simulink model "hdv_ctrl_2021_08_12"  (R2020a)
settings: Solver=ode23tb  StartTime=0.0  StopTime=simulation_length  MaxStep=tsample
values from neighbouring files (symbols this model uses):
  available_torque = [-660.07, -796.01, -907.96, -1019.98, -1070.98, -1123.89,     -1175.99, -1224.03, -1254.98, -1250.99, -1250.98, -1250.98, -1050.04,     -934.05, -780.06, -650, -450, -350, 350, 450, 650, 780.06, 934.05,     1050.04, 1250.98, 1250.98, 1250.99, 1254.98, 1224.03, 1175.99,     1123.89, 1070.98, 1019.98, 907.96, 796.01, 660.07]    [control_design.m]
  d1_ff = d1_ff_temp    (= 1.95205196931)    [control_design.m]
  d2_ff = d2_ff_temp    (= 1.95205196931)    [control_design.m]
  ki_ctrl_diff_speed = 4/n2    (= 4)    [control_design.m]
  ki_ctrl_sum_speed = 4/n1    (= 4)    [control_design.m]
  kp_ctrl_diff_speed = 0.25/n2    (= 0.25)    [control_design.m]
  kp_ctrl_sum_speed = 0.25/n1    (= 0.25)    [control_design.m]
  omega_e_rpm_ref = 1940    [control_design.m]
  omega_l_1_ref_rpm = v_track1_ref/3.6/R_tg/(2*pi)*60    (= 48.1674665855)    [control_design.m]
  omega_l_2_ref_rpm = v_track2_ref/3.6/R_tg/(2*pi)*60    (= 48.1674665855)    [control_design.m]
  omega_l_max_rpm = omega_l_max/(2*pi)*60    (= 66.2302665551)    [control_design.m]
  R_tg = 0.44056    [control_design.m]
  rpm = [-2140, -2100, -2000, -1900, -1800, -1700, -1600, -1500, -1400,          -1300, -1200, -1100, -1000, -900, -800, -700, -600, -5, 5, 600,          700, 800, 900, 1000, 1100, 1200, 1300, 1400, 1500, 1600, 1700, 1800,         1900, 2000, 2100, 2140]    [control_design.m]
  simulation_length = 45    [control_design.m]
  tau_load = -1200*41.4    (= -49680)    [control_design.m]
  tau_load_max = 1600*41.4    (= 66240)    [control_design.m]
  tsample = 1e-3    (= 0.001)    [control_design.m]
  v_track1_ref = 8    [control_design.m]
  v_track2_ref = 8    [control_design.m]
libraries: nesl_utility x24, fl_lib x13, linear_swashplate_ctrl_lib x4, variable_displacement_motor_lib x2, variable_displacement_pump_lib x2, flexshaft_lib x2, gear_lib x2, simulink x2, engine_speed_ctrl_lib x1, Liebherr_Engine_D934_lib x1
settings Model: SimulationMode=accelerator  Creator=dbagn  LastModifiedBy=dbagn
settings DataIOCC: ReturnWorkspaceOutputs=off

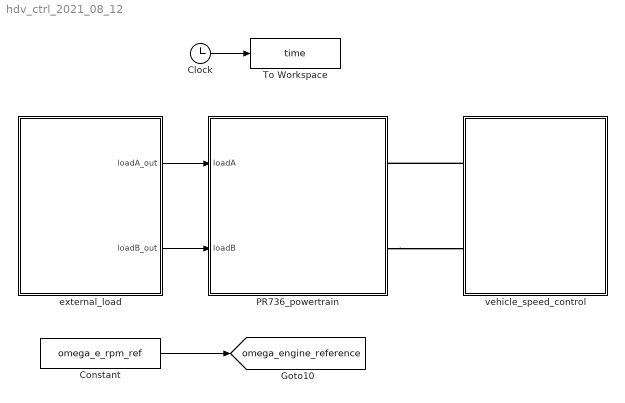
== system hdv_ctrl_2021_08_12 ==
  Clock : Clock
  Constant : Constant  Value=omega_e_rpm_ref
  PR736_powertrain : Subsystem
  To Workspace : ToWorkspace  VariableName=time  SampleTime=tsample
      settings: MaxDataPoints=Nsample
  external_load : Subsystem
  vehicle_speed_control : Subsystem
  tag scope: omega_engine_reference=global
  wires:
  Clock/1 -> To Workspace/1
  Constant/1 -> [omega_engine_reference]
  external_load/2(loadB_out) -> PR736_powertrain/2(loadB)
  external_load/1(loadA_out) -> PR736_powertrain/1(loadA)
  connections:
  vehicle_speed_control/LConn1 -- PR736_powertrain/RConn1
  PR736_powertrain/RConn2 -- vehicle_speed_control/LConn2

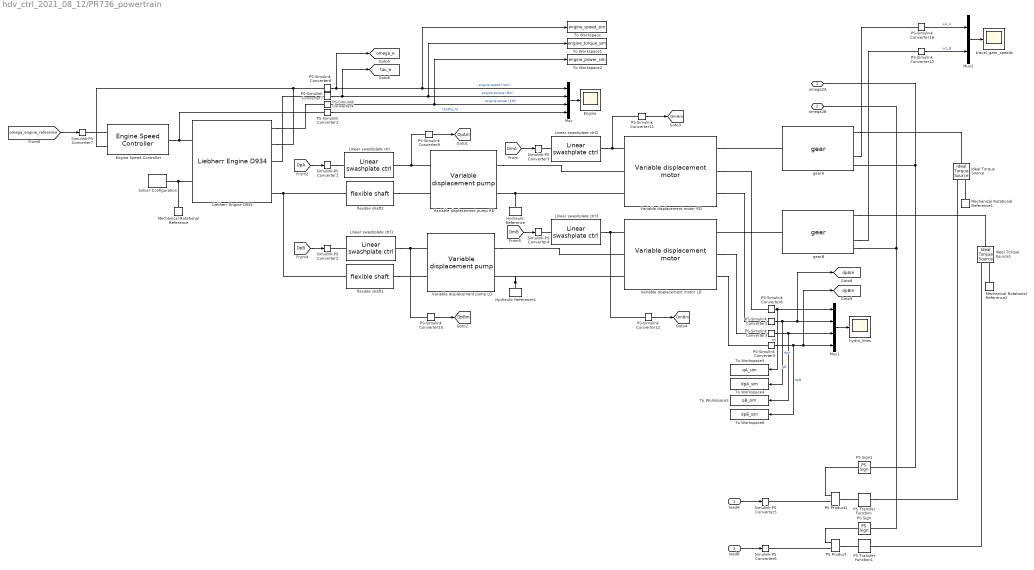
== system hdv_ctrl_2021_08_12/PR736_powertrain ==
  loadA : Inport
  loadB : Inport  Port=2
  Engine : Scope
  Engine Speed Controller : engine_speed_ctrl_lib/Engine Speed Controller  kp=0.25 s  kint=2  kd=0 s^2  t_out_specify=off  t_out_priority=None  t_out=0  t_out_nominal_specify=off  t_out_nominal_unit=1  t_out_nominal_value=1
      settings: InternalSimscapePortConfiguration="{\"Bottom\":[],\"Left\":[{\"id\":\"we_ref\",\"label\":\"we_ref\",\"type\":\"input\"},{\"id\":\"we\",\"label\":\"we\",\"type\":\"input\"}],\"Right\":[{\"id\":\"theta\",\"label\":\"tS\",\"type\":\"output\"}],\"Top\":[]}"
  Hydraulic Reference : fl_lib/Hydraulic/Hydraulic Elements/Hydraulic Reference
  Hydraulic Reference1 : fl_lib/Hydraulic/Hydraulic Elements/Hydraulic Reference
  Ideal Torque Source : fl_lib/Mechanical/Mechanical Sources/Ideal Torque Source
  Ideal Torque Source1 : fl_lib/Mechanical/Mechanical Sources/Ideal Torque Source
  Liebherr Engine D934 : Liebherr_Engine_D934_lib/Liebherr Engine D934  dynamic_response=simscape.enum.onoff.on  cshaft_inertia=7.5 kg*m^2  initial_speed=5
      settings: InternalSimscapePortConfiguration="{\"Bottom\":[],\"Left\":[{\"id\":\"tS\",\"label\":\"tS\",\"type\":\"input\"},{\"id\":\"C\",\"label\":\"C\",\"type\":\"foundation.mechanical.rotational.rotational\"}],\"Right\":[{\"id\":\"PE\",\"label\":\"PE\",\"type\":\"output\"},{\"id\":\"wE\",\"label\":\"wE\",\"type\":\"output\"},{\"id\":\"tE\",\"label\":\"tE\",\"type\":\"output\"},{\"id\":\"eE\",\"label\":\"eE\",\"type\":\"output\"},{\"id\":\"D\",\"label\":\"D\",\"type\":\"foundation.mechanical.rotational.rotational\"}],\"Top\":[]}"
  Linear swashplate ctrl : linear_swashplate_ctrl_lib/Linear swashplate ctrl  a12=1 1/s  b2=1 1/m/s  k1=100 m  k2=20.5 m  N=10 m  kv=10  xv_specify=off  xv_priority=None  xv=0 m  xv_nominal_specify=off  xv_nominal_unit=m  xv_nominal_value=1  D1_specify=off  D1_priority=None  D1=0  D1_nominal_specify=off  D1_nominal_unit=1  D1_nominal_value=1  D2_specify=off  D2_priority=None  D2=0  D2_nominal_specify=off  D2_nominal_unit=1  D2_nominal_value=1
      settings: InternalSimscapePortConfiguration="{\"Bottom\":[],\"Left\":[{\"id\":\"D_ref\",\"label\":\"Dref\",\"type\":\"input\"}],\"Right\":[{\"id\":\"Dout\",\"label\":\"Dout\",\"type\":\"output\"}],\"Top\":[]}"
  Linear swashplate ctrl1 : linear_swashplate_ctrl_lib/Linear swashplate ctrl  a12=1 1/s  b2=1 1/m/s  k1=100 m  k2=20.5 m  N=10 m  kv=10  xv_specify=off  xv_priority=None  xv=0 m  xv_nominal_specify=off  xv_nominal_unit=m  xv_nominal_value=1  D1_specify=off  D1_priority=None  D1=0  D1_nominal_specify=off  D1_nominal_unit=1  D1_nominal_value=1  D2_specify=off  D2_priority=None  D2=0  D2_nominal_specify=off  D2_nominal_unit=1  D2_nominal_value=1
      settings: InternalSimscapePortConfiguration="{\"Bottom\":[],\"Left\":[{\"id\":\"D_ref\",\"label\":\"Dref\",\"type\":\"input\"}],\"Right\":[{\"id\":\"Dout\",\"label\":\"Dout\",\"type\":\"output\"}],\"Top\":[]}"
  Linear swashplate ctrl2 : linear_swashplate_ctrl_lib/Linear swashplate ctrl  a12=1 1/s  b2=1 1/m/s  k1=100 m  k2=20.5 m  N=5 m  kv=20  xv_specify=off  xv_priority=None  xv=0 m  xv_nominal_specify=off  xv_nominal_unit=m  xv_nominal_value=1  D1_specify=off  D1_priority=None  D1=0  D1_nominal_specify=off  D1_nominal_unit=1  D1_nominal_value=1  D2_specify=off  D2_priority=None  D2=0  D2_nominal_specify=off  D2_nominal_unit=1  D2_nominal_value=1
      settings: InternalSimscapePortConfiguration="{\"Bottom\":[],\"Left\":[{\"id\":\"D_ref\",\"label\":\"Dref\",\"type\":\"input\"}],\"Right\":[{\"id\":\"Dout\",\"label\":\"Dout\",\"type\":\"output\"}],\"Top\":[]}"
  Linear swashplate ctrl3 : linear_swashplate_ctrl_lib/Linear swashplate ctrl  a12=1 1/s  b2=1 1/m/s  k1=100 m  k2=20.5 m  N=5 m  kv=20  xv_specify=off  xv_priority=None  xv=0 m  xv_nominal_specify=off  xv_nominal_unit=m  xv_nominal_value=1  D1_specify=off  D1_priority=None  D1=0  D1_nominal_specify=off  D1_nominal_unit=1  D1_nominal_value=1  D2_specify=off  D2_priority=None  D2=0  D2_nominal_specify=off  D2_nominal_unit=1  D2_nominal_value=1
      settings: InternalSimscapePortConfiguration="{\"Bottom\":[],\"Left\":[{\"id\":\"D_ref\",\"label\":\"Dref\",\"type\":\"input\"}],\"Right\":[{\"id\":\"Dout\",\"label\":\"Dout\",\"type\":\"output\"}],\"Top\":[]}"
  Mechanical Rotational Reference : fl_lib/Mechanical/Rotational Elements/Mechanical Rotational Reference
  Mechanical Rotational Reference1 : fl_lib/Mechanical/Rotational Elements/Mechanical Rotational Reference
  Mechanical Rotational Reference2 : fl_lib/Mechanical/Rotational Elements/Mechanical Rotational Reference
  Mux : Mux
  Mux1 : Mux
  Mux2 : Mux  Inputs=2
  PS Product : fl_lib/Physical Signals/Functions/PS Product
  PS Product1 : fl_lib/Physical Signals/Functions/PS Product
  PS Sign : fl_lib/Physical Signals/Nonlinear Operators/PS Sign
      settings: SourceProductBaseCode=SS  InternalSimscapePortConfiguration="{\"Bottom\":[],\"Left\":[{\"id\":\"I\",\"label\":\"\",\"type\":\"input\"}],\"Right\":[{\"id\":\"O\",\"label\":\"\",\"type\":\"output\"}],\"Top\":[]}"
  PS Sign1 : fl_lib/Physical Signals/Nonlinear Operators/PS Sign
      settings: SourceProductBaseCode=SS  InternalSimscapePortConfiguration="{\"Bottom\":[],\"Left\":[{\"id\":\"I\",\"label\":\"\",\"type\":\"input\"}],\"Right\":[{\"id\":\"O\",\"label\":\"\",\"type\":\"output\"}],\"Top\":[]}"
  PS Transfer Function : fl_lib/Physical Signals/Linear Operators/PS Transfer Function  transfer_function_type=foundation.enum.transfer_function_type.lag  T=1 s  T1=2 s  T2=1 s  y0=0 N*m
      settings: SourceProductBaseCode=SS  InternalSimscapePortConfiguration="{\"Bottom\":[],\"Left\":[{\"id\":\"U\",\"label\":\"\",\"type\":\"input\"}],\"Right\":[{\"id\":\"Y\",\"label\":\"\",\"type\":\"output\"}],\"Top\":[]}"
  PS Transfer Function1 : fl_lib/Physical Signals/Linear Operators/PS Transfer Function  transfer_function_type=foundation.enum.transfer_function_type.lag  T=1 s  T1=2 s  T2=1 s  y0=0 N*m
      settings: SourceProductBaseCode=SS  InternalSimscapePortConfiguration="{\"Bottom\":[],\"Left\":[{\"id\":\"U\",\"label\":\"\",\"type\":\"input\"}],\"Right\":[{\"id\":\"Y\",\"label\":\"\",\"type\":\"output\"}],\"Top\":[]}"
  PS-Simulink Converter1 : nesl_utility/PS-Simulink Converter  PhysicalDomain=network_engine_domain  SubClassName=ps_output  LeftPortType=input  RightPortType=output  PseudoPeriodic=off  Frequencies=[]  Unit=inherit  AffineConversion=off
  PS-Simulink Converter{2,5,9..12} (6 alike) : nesl_utility/PS-Simulink Converter  PhysicalDomain=network_engine_domain  SubClassName=ps_output  LeftPortType=input  RightPortType=output  PseudoPeriodic=off  Frequencies=[]  Unit=bar  AffineConversion=off
  PS-Simulink Converter13 : nesl_utility/PS-Simulink Converter  PhysicalDomain=network_engine_domain  SubClassName=ps_output  LeftPortType=input  RightPortType=output  PseudoPeriodic=off  Frequencies=[]  Unit=rpm  AffineConversion=on
  PS-Simulink Converter16 : nesl_utility/PS-Simulink Converter  PhysicalDomain=network_engine_domain  SubClassName=ps_output  LeftPortType=input  RightPortType=output  PseudoPeriodic=off  Frequencies=[]  Unit=rpm  AffineConversion=on
  PS-Simulink Converter3 : nesl_utility/PS-Simulink Converter  PhysicalDomain=network_engine_domain  SubClassName=ps_output  LeftPortType=input  RightPortType=output  PseudoPeriodic=off  Frequencies=[]  Unit=l/min  AffineConversion=off
  PS-Simulink Converter4 : nesl_utility/PS-Simulink Converter  PhysicalDomain=network_engine_domain  SubClassName=ps_output  LeftPortType=input  RightPortType=output  PseudoPeriodic=off  Frequencies=[]  Unit=kW  AffineConversion=off
  PS-Simulink Converter6 : nesl_utility/PS-Simulink Converter  PhysicalDomain=network_engine_domain  SubClassName=ps_output  LeftPortType=input  RightPortType=output  PseudoPeriodic=off  Frequencies=[]  Unit=rpm  AffineConversion=off
  PS-Simulink Converter7 : nesl_utility/PS-Simulink Converter  PhysicalDomain=network_engine_domain  SubClassName=ps_output  LeftPortType=input  RightPortType=output  PseudoPeriodic=off  Frequencies=[]  Unit=inherit  AffineConversion=off
  PS-Simulink Converter8 : nesl_utility/PS-Simulink Converter  PhysicalDomain=network_engine_domain  SubClassName=ps_output  LeftPortType=input  RightPortType=output  PseudoPeriodic=off  Frequencies=[]  Unit=l/min  AffineConversion=off
  Simulink-PS Converter{1..4} (4 alike) : nesl_utility/Simulink-PS Converter  PhysicalDomain=network_engine_domain  SubClassName=ps_input  LeftPortType=input  RightPortType=output  PseudoPeriodic=off  Frequencies=[]  NoiseDistribution=none  NoiseParameters=[]  Unit=1  AffineConversion=off  FilteringAndDerivatives=provide  SimscapeFilterOrder=1  InputFilterTimeConstant=0.001  UdotUserProvided=0
  Simulink-PS Converter5 : nesl_utility/Simulink-PS Converter  PhysicalDomain=network_engine_domain  SubClassName=ps_input  LeftPortType=input  RightPortType=output  PseudoPeriodic=off  Frequencies=[]  NoiseDistribution=none  NoiseParameters=[]  Unit=N*m  AffineConversion=off  FilteringAndDerivatives=provide  SimscapeFilterOrder=1  InputFilterTimeConstant=0.001  UdotUserProvided=0
  Simulink-PS Converter6 : nesl_utility/Simulink-PS Converter  PhysicalDomain=network_engine_domain  SubClassName=ps_input  LeftPortType=input  RightPortType=output  PseudoPeriodic=off  Frequencies=[]  NoiseDistribution=none  NoiseParameters=[]  Unit=N*m  AffineConversion=off  FilteringAndDerivatives=provide  SimscapeFilterOrder=1  InputFilterTimeConstant=0.001  UdotUserProvided=0
  Simulink-PS Converter7 : nesl_utility/Simulink-PS Converter  PhysicalDomain=network_engine_domain  SubClassName=ps_input  LeftPortType=input  RightPortType=output  PseudoPeriodic=off  Frequencies=[]  NoiseDistribution=none  NoiseParameters=[]  Unit=rpm  AffineConversion=off  FilteringAndDerivatives=provide  SimscapeFilterOrder=1  InputFilterTimeConstant=0.001  UdotUserProvided=0
  Solver Configuration : nesl_utility/Solver Configuration  PhysicalDomain=network_engine_domain  SubClassName=solver  LeftPortType=input  RightPortType=generic  Tones=[]  Harmonics=[]  SimulateNoise=off  Profile=off  UseLocalSampling=off  EnableSwitchedLinearOptims=on  FrequencyDomain=off  UseCCode=off  RelTol=0.001  AbsTol=1e-06  MinStep=1e-09  ToWorkspace=off  RevertToSquareIcSolve=off  NumHomotopyIterations=100  PhasorMode=off  PhasorModeNumHarmonics=1  DoDC=off  ResidualTolerance=1e-09  UseLocalSolver=on  LocalSolverChoice=NE_BACKWARD_EULER_ADVANCER  LocalSolverSampleTime=tsample  DoFixedCost=on  MaxNonlinIter=3  MaxModeIter=2  LinearAlgebra=auto  EquationFormulation=NE_TIME_EF  DelaysMemoryBudget=1024  AutomaticFiltering=on  FilteringTimeConstant=tsample  PartitionStorageMethod=AS_NEEDED  PartitionMemoryBudget=1024  PartitionMethod=ROBUST
  To Workspace : ToWorkspace  VariableName=engine_speed_sim  SampleTime=tsample
      settings: MaxDataPoints=Nsample
  To Workspace1 : ToWorkspace  VariableName=engine_torque_sim  SampleTime=tsample
      settings: MaxDataPoints=Nsample
  To Workspace2 : ToWorkspace  VariableName=engine_power_sim  SampleTime=tsample
      settings: MaxDataPoints=Nsample
  To Workspace3 : ToWorkspace  VariableName=qA_sim  SampleTime=tsample
      settings: MaxDataPoints=Nsample
  To Workspace4 : ToWorkspace  VariableName=dpA_sim  SampleTime=tsample
      settings: MaxDataPoints=Nsample
  To Workspace5 : ToWorkspace  VariableName=qB_sim  SampleTime=tsample
      settings: MaxDataPoints=Nsample
  To Workspace6 : ToWorkspace  VariableName=dpB_sim  SampleTime=tsample
      settings: MaxDataPoints=Nsample
  Variable displacement motor LD : variable_displacement_motor_lib/Variable displacement motor  max_Dv=Vm_nom cm^3/rev  min_Dv=20 cm^3/rev  inertia_motor=0.0402 kg*m^2  oil_vol=4.1 l  eta_mech=eta_m_m  eta_vol=eta_v_m  t_specify=off  t_priority=None  t=0 N*m  t_nominal_specify=off  t_nominal_unit=N*m  t_nominal_value=1  q_specify=off  q_priority=None  q=0 m^3/s  q_nominal_specify=off  q_nominal_unit=m^3/s  q_nominal_value=1  qt_specify=off  qt_priority=None  qt=0 m^3/s  qt_nominal_specify=off  qt_nominal_unit=m^3/s  qt_nominal_value=1  Dv_specify=off  Dv_priority=None  Dv=0 cm^3/rev  Dv_nominal_specify=off  Dv_nominal_unit=cm^3/rev  Dv_nominal_value=1  dp_specify=off  dp_priority=None  dp=0 Pa  dp_nominal_specify=off  dp_nominal_unit=Pa  dp_nominal_value=1  wm_specify=off  wm_priority=None  wm=0 rad/s  wm_nominal_specify=off  wm_nominal_unit=rad/s  wm_nominal_value=1
      settings: InternalSimscapePortConfiguration="{\"Bottom\":[],\"Left\":[{\"id\":\"Vd\",\"label\":\"Vd\",\"type\":\"input\"},{\"id\":\"A\",\"label\":\"A\",\"type\":\"foundation.hydraulic.hydraulic\"},{\"id\":\"B\",\"label\":\"B\",\"type\":\"foundation.hydraulic.hydraulic\"}],\"Right\":[{\"id\":\"C\",\"label\":\"C\",\"type\":\"foundation.mechanical.rotational.rotational\"},{\"id\":\"q_out\",\"label\":\"q\",\"type\":\"output\"},{\"id\":\"delta_p_out\",\"label\":\"delta_p\",\"type\":\"output\"}],\"Top\":[]}"
  Variable displacement motor RD : variable_displacement_motor_lib/Variable displacement motor  max_Dv=Vm_nom cm^3/rev  min_Dv=20 cm^3/rev  inertia_motor=0.0402 kg*m^2  oil_vol=4.1 l  eta_mech=eta_m_m  eta_vol=eta_v_m  t_specify=off  t_priority=None  t=0 N*m  t_nominal_specify=off  t_nominal_unit=N*m  t_nominal_value=1  q_specify=off  q_priority=None  q=0 m^3/s  q_nominal_specify=off  q_nominal_unit=m^3/s  q_nominal_value=1  qt_specify=off  qt_priority=None  qt=0 m^3/s  qt_nominal_specify=off  qt_nominal_unit=m^3/s  qt_nominal_value=1  Dv_specify=off  Dv_priority=None  Dv=0 cm^3/rev  Dv_nominal_specify=off  Dv_nominal_unit=cm^3/rev  Dv_nominal_value=1  dp_specify=off  dp_priority=None  dp=0 Pa  dp_nominal_specify=off  dp_nominal_unit=Pa  dp_nominal_value=1  wm_specify=off  wm_priority=None  wm=0 rad/s  wm_nominal_specify=off  wm_nominal_unit=rad/s  wm_nominal_value=1
      settings: InternalSimscapePortConfiguration="{\"Bottom\":[],\"Left\":[{\"id\":\"Vd\",\"label\":\"Vd\",\"type\":\"input\"},{\"id\":\"A\",\"label\":\"A\",\"type\":\"foundation.hydraulic.hydraulic\"},{\"id\":\"B\",\"label\":\"B\",\"type\":\"foundation.hydraulic.hydraulic\"}],\"Right\":[{\"id\":\"C\",\"label\":\"C\",\"type\":\"foundation.mechanical.rotational.rotational\"},{\"id\":\"q_out\",\"label\":\"q\",\"type\":\"output\"},{\"id\":\"delta_p_out\",\"label\":\"delta_p\",\"type\":\"output\"}],\"Top\":[]}"
  Variable displacement pump LD : variable_displacement_pump_lib/Variable displacement pump  max_Dv=Vp_nom cm^3/rev  inertia_pump=0.027 kg*m^2  oil_vol=3.0 l  eta_mech=eta_m_p  eta_vol=eta_v_p  t_specify=off  t_priority=None  t=0 N*m  t_nominal_specify=off  t_nominal_unit=N*m  t_nominal_value=1  q_specify=off  q_priority=None  q=0 m^3/s  q_nominal_specify=off  q_nominal_unit=m^3/s  q_nominal_value=1  qt_specify=off  qt_priority=None  qt=0 m^3/s  qt_nominal_specify=off  qt_nominal_unit=m^3/s  qt_nominal_value=1  Dv_specify=off  Dv_priority=None  Dv=0 cm^3/rev  Dv_nominal_specify=off  Dv_nominal_unit=cm^3/rev  Dv_nominal_value=1  dp_specify=off  dp_priority=None  dp=0 Pa  dp_nominal_specify=off  dp_nominal_unit=Pa  dp_nominal_value=1  we_specify=off  we_priority=None  we=0 rad/s  we_nominal_specify=off  we_nominal_unit=rad/s  we_nominal_value=1
      settings: InternalSimscapePortConfiguration="{\"Bottom\":[],\"Left\":[{\"id\":\"Vd\",\"label\":\"Vd\",\"type\":\"input\"},{\"id\":\"C\",\"label\":\"C\",\"type\":\"foundation.mechanical.rotational.rotational\"}],\"Right\":[{\"id\":\"A\",\"label\":\"A\",\"type\":\"foundation.hydraulic.hydraulic\"},{\"id\":\"B\",\"label\":\"B\",\"type\":\"foundation.hydraulic.hydraulic\"}],\"Top\":[]}"
  Variable displacement pump RD : variable_displacement_pump_lib/Variable displacement pump  max_Dv=Vp_nom cm^3/rev  inertia_pump=0.027 kg*m^2  oil_vol=3.0 l  eta_mech=eta_m_p  eta_vol=eta_v_p  t_specify=off  t_priority=None  t=0 N*m  t_nominal_specify=off  t_nominal_unit=N*m  t_nominal_value=1  q_specify=off  q_priority=None  q=0 m^3/s  q_nominal_specify=off  q_nominal_unit=m^3/s  q_nominal_value=1  qt_specify=off  qt_priority=None  qt=0 m^3/s  qt_nominal_specify=off  qt_nominal_unit=m^3/s  qt_nominal_value=1  Dv_specify=off  Dv_priority=None  Dv=0 cm^3/rev  Dv_nominal_specify=off  Dv_nominal_unit=cm^3/rev  Dv_nominal_value=1  dp_specify=off  dp_priority=None  dp=0 Pa  dp_nominal_specify=off  dp_nominal_unit=Pa  dp_nominal_value=1  we_specify=off  we_priority=None  we=0 rad/s  we_nominal_specify=off  we_nominal_unit=rad/s  we_nominal_value=1
      settings: InternalSimscapePortConfiguration="{\"Bottom\":[],\"Left\":[{\"id\":\"Vd\",\"label\":\"Vd\",\"type\":\"input\"},{\"id\":\"C\",\"label\":\"C\",\"type\":\"foundation.mechanical.rotational.rotational\"}],\"Right\":[{\"id\":\"A\",\"label\":\"A\",\"type\":\"foundation.hydraulic.hydraulic\"},{\"id\":\"B\",\"label\":\"B\",\"type\":\"foundation.hydraulic.hydraulic\"}],\"Top\":[]}"
  flexible shaft1 : flexshaft_lib/flexible shaft  b1=b1 N*m/(rad/s)  J1=J1 kg*m^2  b2=b2 N*m/(rad/s)  J2=J2 kg*m^2  b_theta=b_theta N*m/(rad/s)  k_theta=k_theta N*m/rad  w_1_specify=off  w_1_priority=None  w_1=0 rad/s  w_1_nominal_specify=off  w_1_nominal_unit=rad/s  w_1_nominal_value=1  w_2_specify=off  w_2_priority=None  w_2=0 rad/s  w_2_nominal_specify=off  w_2_nominal_unit=rad/s  w_2_nominal_value=1  t_1_specify=off  t_1_priority=None  t_1=0 N*m  t_1_nominal_specify=off  t_1_nominal_unit=N*m  t_1_nominal_value=1  t_2_specify=off  t_2_priority=None  t_2=0 N*m  t_2_nominal_specify=off  t_2_nominal_unit=N*m  t_2_nominal_value=1  t_theta_specify=off  t_theta_priority=None  t_theta=0 N*m  t_theta_nominal_specify=off  t_theta_nominal_unit=N*m  t_theta_nominal_value=1
      settings: InternalSimscapePortConfiguration="{\"Bottom\":[],\"Left\":[{\"id\":\"S1\",\"label\":\"S1\",\"type\":\"foundation.mechanical.rotational.rotational\"}],\"Right\":[{\"id\":\"S2\",\"label\":\"S2\",\"type\":\"foundation.mechanical.rotational.rotational\"}],\"Top\":[]}"
  flexible shaft2 : flexshaft_lib/flexible shaft  b1=b1 N*m/(rad/s)  J1=J1 kg*m^2  b2=b2 N*m/(rad/s)  J2=J2 kg*m^2  b_theta=b_theta N*m/(rad/s)  k_theta=k_theta N*m/rad  w_1_specify=off  w_1_priority=None  w_1=0 rad/s  w_1_nominal_specify=off  w_1_nominal_unit=rad/s  w_1_nominal_value=1  w_2_specify=off  w_2_priority=None  w_2=0 rad/s  w_2_nominal_specify=off  w_2_nominal_unit=rad/s  w_2_nominal_value=1  t_1_specify=off  t_1_priority=None  t_1=0 N*m  t_1_nominal_specify=off  t_1_nominal_unit=N*m  t_1_nominal_value=1  t_2_specify=off  t_2_priority=None  t_2=0 N*m  t_2_nominal_specify=off  t_2_nominal_unit=N*m  t_2_nominal_value=1  t_theta_specify=off  t_theta_priority=None  t_theta=0 N*m  t_theta_nominal_specify=off  t_theta_nominal_unit=N*m  t_theta_nominal_value=1
      settings: InternalSimscapePortConfiguration="{\"Bottom\":[],\"Left\":[{\"id\":\"S1\",\"label\":\"S1\",\"type\":\"foundation.mechanical.rotational.rotational\"}],\"Right\":[{\"id\":\"S2\",\"label\":\"S2\",\"type\":\"foundation.mechanical.rotational.rotational\"}],\"Top\":[]}"
  gearA : gear_lib/gear  n1=n_tg  n2=1  b1=0.02 N*m/(rad/s)  J1=0.25 kg*m^2  b2=track_friction_1 N*m/(rad/s)  J2=2 kg*m^2  k_theta_1=k_theta N*m/rad  w_1_specify=off  w_1_priority=None  w_1=0 rad/s  w_1_nominal_specify=off  w_1_nominal_unit=rad/s  w_1_nominal_value=1  w_2_specify=off  w_2_priority=None  w_2=0 rad/s  w_2_nominal_specify=off  w_2_nominal_unit=rad/s  w_2_nominal_value=1  t_1_specify=off  t_1_priority=None  t_1=0 N*m  t_1_nominal_specify=off  t_1_nominal_unit=N*m  t_1_nominal_value=1  t_2_specify=off  t_2_priority=None  t_2=0 N*m  t_2_nominal_specify=off  t_2_nominal_unit=N*m  t_2_nominal_value=1  t_theta_1_specify=off  t_theta_1_priority=None  t_theta_1=0 N*m  t_theta_1_nominal_specify=off  t_theta_1_nominal_unit=N*m  t_theta_1_nominal_value=1  t_theta_2_specify=off  t_theta_2_priority=None  t_theta_2=0 N*m  t_theta_2_nominal_specify=off  t_theta_2_nominal_unit=N*m  t_theta_2_nominal_value=1
      settings: InternalSimscapePortConfiguration="{\"Bottom\":[],\"Left\":[{\"id\":\"S1\",\"label\":\"S1\",\"type\":\"foundation.mechanical.rotational.rotational\"}],\"Right\":[{\"id\":\"S2\",\"label\":\"S2\",\"type\":\"foundation.mechanical.rotational.rotational\"},{\"id\":\"tau_theta_1\",\"label\":\"tau_theta_1\",\"type\":\"output\"},{\"id\":\"tau_theta_2\",\"label\":\"tau_theta_2\",\"type\":\"output\"},{\"id\":\"w1\",\"label\":\"w1\",\"type\":\"output\"},{\"id\":\"w2\",\"label\":\"w2\",\"type\":\"output\"}],\"Top\":[]}"
  gearB : gear_lib/gear  n1=n_tg  n2=1  b1=0.02 N*m/(rad/s)  J1=0.25 kg*m^2  b2=track_friction_2 N*m/(rad/s)  J2=2 kg*m^2  k_theta_1=k_theta N*m/rad  w_1_specify=off  w_1_priority=None  w_1=0 rad/s  w_1_nominal_specify=off  w_1_nominal_unit=rad/s  w_1_nominal_value=1  w_2_specify=off  w_2_priority=None  w_2=0 rad/s  w_2_nominal_specify=off  w_2_nominal_unit=rad/s  w_2_nominal_value=1  t_1_specify=off  t_1_priority=None  t_1=0 N*m  t_1_nominal_specify=off  t_1_nominal_unit=N*m  t_1_nominal_value=1  t_2_specify=off  t_2_priority=None  t_2=0 N*m  t_2_nominal_specify=off  t_2_nominal_unit=N*m  t_2_nominal_value=1  t_theta_1_specify=off  t_theta_1_priority=None  t_theta_1=0 N*m  t_theta_1_nominal_specify=off  t_theta_1_nominal_unit=N*m  t_theta_1_nominal_value=1  t_theta_2_specify=off  t_theta_2_priority=None  t_theta_2=0 N*m  t_theta_2_nominal_specify=off  t_theta_2_nominal_unit=N*m  t_theta_2_nominal_value=1
      settings: InternalSimscapePortConfiguration="{\"Bottom\":[],\"Left\":[{\"id\":\"S1\",\"label\":\"S1\",\"type\":\"foundation.mechanical.rotational.rotational\"}],\"Right\":[{\"id\":\"S2\",\"label\":\"S2\",\"type\":\"foundation.mechanical.rotational.rotational\"},{\"id\":\"tau_theta_1\",\"label\":\"tau_theta_1\",\"type\":\"output\"},{\"id\":\"tau_theta_2\",\"label\":\"tau_theta_2\",\"type\":\"output\"},{\"id\":\"w1\",\"label\":\"w1\",\"type\":\"output\"},{\"id\":\"w2\",\"label\":\"w2\",\"type\":\"output\"}],\"Top\":[]}"
  hydro_lines : Scope
  travel_gear_speeds : Scope
  omega2A : PMIOPort  Side=Right
  omega2B : PMIOPort  Port=2  Side=Right
  tag scope: DmAm=global, DmBm=global, DpAm=global, DpBm=global, dpAm=global, dpBm=global, omega_e=global, tau_e=global
  wires:
  PS-Simulink Converter7/1 -> [tau_e], To Workspace1/1, Mux/2  "engine torque (Nm)"
  Mux1/1 -> hydro_lines/1
  PS-Simulink Converter5/1 -> To Workspace6/1, Mux1/4, [dpBm]  "dpB"
  PS-Simulink Converter8/1 -> To Workspace3/1, Mux1/1  "qA"
  [DmB] -> Simulink-PS Converter4/1
  PS-Simulink Converter6/1 -> [omega_e], To Workspace/1, Mux/1  "engine speed (rpm)"
  PS-Simulink Converter3/1 -> To Workspace5/1, Mux1/3  "qB"
  Mux/1 -> Engine/1
  [DpA] -> Simulink-PS Converter1/1
  PS-Simulink Converter2/1 -> To Workspace4/1, Mux1/2, [dpAm]  "dpA"
  [DmA] -> Simulink-PS Converter3/1
  [DpB] -> Simulink-PS Converter2/1
  PS-Simulink Converter1/1 -> Mux/4  "thottle_%"
  PS-Simulink Converter4/1 -> Mux/3, To Workspace2/1  "engine power (kW)"
  PS-Simulink Converter10/1 -> [DpBm]
  PS-Simulink Converter9/1 -> [DpAm]
  PS-Simulink Converter11/1 -> [DmAm]
  PS-Simulink Converter12/1 -> [DmBm]
  [omega_engine_reference] -> Simulink-PS Converter7/1
  loadA/1 -> Simulink-PS Converter5/1
  loadB/1 -> Simulink-PS Converter6/1
  PS-Simulink Converter13/1 -> Mux2/2  "w1_B"
  PS-Simulink Converter16/1 -> Mux2/1  "w1_A"
  Mux2/1 -> travel_gear_speeds/1
  connections:
  Engine Speed Controller/RConn1 -- PS-Simulink Converter1/LConn1 -- Liebherr Engine D934/LConn1
  Liebherr Engine D934/RConn1 -- PS-Simulink Converter4/LConn1
  Linear swashplate ctrl1/LConn1 -- Simulink-PS Converter2/RConn1
  Linear swashplate ctrl1/RConn1 -- PS-Simulink Converter10/LConn1 -- Variable displacement pump LD/LConn1
  Variable displacement pump RD/RConn1 -- Variable displacement motor RD/LConn2
  Simulink-PS Converter7/RConn1 -- Engine Speed Controller/LConn1
  Liebherr Engine D934/RConn2 -- Engine Speed Controller/LConn2 -- PS-Simulink Converter6/LConn1
  Variable displacement pump LD/RConn1 -- Variable displacement motor LD/LConn2
  flexible shaft1/RConn1 -- Variable displacement pump LD/LConn2
  Liebherr Engine D934/LConn2 -- Mechanical Rotational Reference/LConn1 -- Solver Configuration/RConn1
  Mechanical Rotational Reference1/LConn1 -- Ideal Torque Source/RConn2
  flexible shaft2/RConn1 -- Variable displacement pump RD/LConn2
  Hydraulic Reference1/LConn1 -- Variable displacement pump LD/RConn2 -- Variable displacement motor LD/LConn3
  Liebherr Engine D934/RConn5 -- flexible shaft2/LConn1 -- flexible shaft1/LConn1
  PS Sign1/RConn1 -- PS Product1/LConn1
  Linear swashplate ctrl3/RConn1 -- Variable displacement motor LD/LConn1 -- PS-Simulink Converter12/LConn1
  Linear swashplate ctrl/RConn1 -- PS-Simulink Converter9/LConn1 -- Variable displacement pump RD/LConn1
  gearB/LConn1 -- Variable displacement motor LD/RConn1
  Variable displacement motor LD/RConn2 -- PS-Simulink Converter3/LConn1
  Linear swashplate ctrl2/RConn1 -- Variable displacement motor RD/LConn1 -- PS-Simulink Converter11/LConn1
  Variable displacement motor RD/LConn3 -- Hydraulic Reference/LConn1 -- Variable displacement pump RD/RConn2
  Linear swashplate ctrl3/LConn1 -- Simulink-PS Converter4/RConn1
  Simulink-PS Converter1/RConn1 -- Linear swashplate ctrl/LConn1
  gearB/RConn5 -- omega2B/RConn1 -- PS Sign/LConn1
  Variable displacement motor RD/RConn3 -- PS-Simulink Converter2/LConn1
  PS-Simulink Converter7/LConn1 -- Liebherr Engine D934/RConn3
  Mechanical Rotational Reference2/LConn1 -- Ideal Torque Source1/RConn2
  PS Product/LConn2 -- Simulink-PS Converter6/RConn1
  PS Transfer Function/RConn1 -- Ideal Torque Source/RConn1
  omega2A/RConn1 -- gearA/RConn5 -- PS Sign1/LConn1
  PS Product/RConn1 -- PS Transfer Function1/LConn1
  PS Sign/RConn1 -- PS Product/LConn1
  Simulink-PS Converter3/RConn1 -- Linear swashplate ctrl2/LConn1
  Variable displacement motor RD/RConn1 -- gearA/LConn1
  Variable displacement motor LD/RConn3 -- PS-Simulink Converter5/LConn1
  Variable displacement motor RD/RConn2 -- PS-Simulink Converter8/LConn1
  PS Product1/RConn1 -- PS Transfer Function/LConn1
  PS Transfer Function1/RConn1 -- Ideal Torque Source1/RConn1
  PS Product1/LConn2 -- Simulink-PS Converter5/RConn1
  gearB/RConn4 -- PS-Simulink Converter13/LConn1
  gearA/RConn4 -- PS-Simulink Converter16/LConn1
  gearA/RConn1 -- Ideal Torque Source/LConn1
  gearB/RConn1 -- Ideal Torque Source1/LConn1

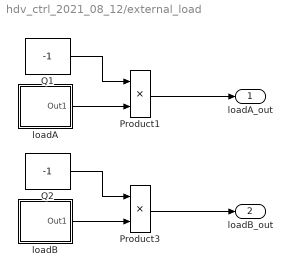
== system hdv_ctrl_2021_08_12/external_load ==
  Product1 : Product
  Product3 : Product
  Q1 : Constant  Value=-1
  Q2 : Constant  Value=-1
  loadA : Subsystem
  loadB : Subsystem
  loadA_out : Outport
  loadB_out : Outport  Port=2
  wires:
  Product1/1 -> loadA_out/1
  loadB/1(Out1) -> Product3/2
  loadA/1(Out1) -> Product1/2
  Q2/1 -> Product3/1
  Product3/1 -> loadB_out/1
  Q1/1 -> Product1/1

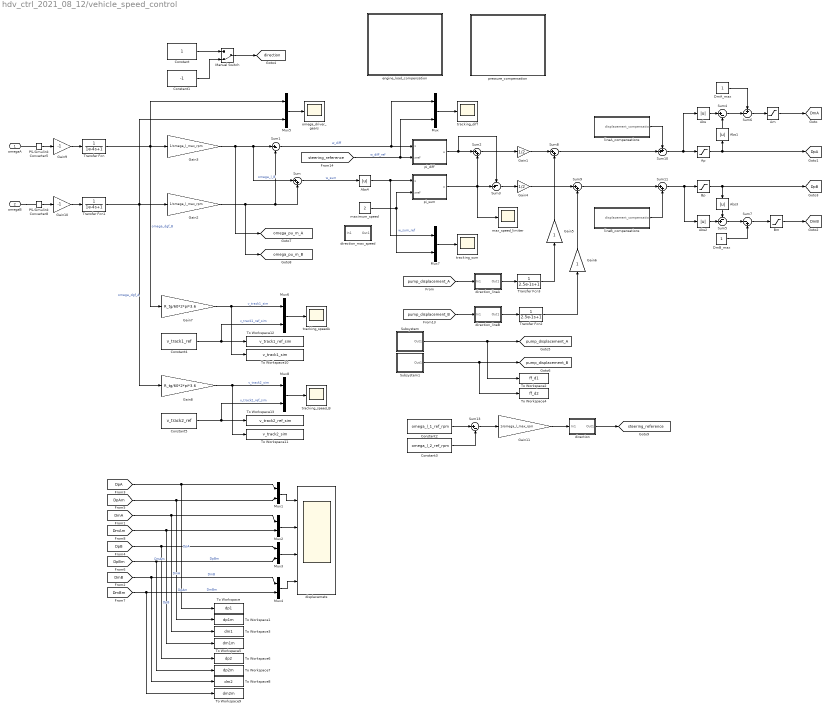
== system hdv_ctrl_2021_08_12/vehicle_speed_control ==
  Abs{,1..4} (5 alike) : Abs
  Am : Saturate  UpperLimit=1  LowerLimit=0.2
  Ap : Saturate  UpperLimit=1  LowerLimit=-1
  Bm : Saturate  UpperLimit=1  LowerLimit=0.2
  Bp : Saturate  UpperLimit=1  LowerLimit=-1
  Constant : Constant
  Constant1 : Constant  Value=-1
  Constant2 : Constant  Value=omega_l_1_ref_rpm
  Constant3 : Constant  Value=omega_l_2_ref_rpm
  Constant4 : Constant  Value=v_track1_ref
  Constant5 : Constant  Value=v_track2_ref
  DmA_max : Constant
  DmB_max : Constant
  Gain1 : Gain  Gain=1/2
  Gain10 : Gain  Gain=-1
  Gain11 : Gain  Gain=1/omega_l_max_rpm
  Gain2 : Gain  Gain=1/omega_l_max_rpm
  Gain3 : Gain  Gain=1/omega_l_max_rpm
  Gain4 : Gain  Gain=1/2
  Gain5 : Gain
  Gain6 : Gain
  Gain7 : Gain  Gain=R_tg/60*2*pi*3.6
  Gain8 : Gain  Gain=R_tg/60*2*pi*3.6
  Gain9 : Gain  Gain=-1
  Manual Switch : ManualSwitch  CurrentSetting=0
  Mux{,1..8} (9 alike) : Mux  Inputs=2
  PS-Simulink Converter5 : nesl_utility/PS-Simulink Converter  PhysicalDomain=network_engine_domain  SubClassName=ps_output  LeftPortType=input  RightPortType=output  PseudoPeriodic=off  Frequencies=[]  Unit=rpm  AffineConversion=off
  PS-Simulink Converter8 : nesl_utility/PS-Simulink Converter  PhysicalDomain=network_engine_domain  SubClassName=ps_output  LeftPortType=input  RightPortType=output  PseudoPeriodic=off  Frequencies=[]  Unit=rpm  AffineConversion=off
  Subsystem : Subsystem
  Subsystem1 : Subsystem
  Sum{,2,8..9,11} (5 alike) : Sum  Inputs=|++
  Sum1 : Sum  Inputs=|+-
  Sum10 : Sum  Inputs=++|
  Sum13 : Sum  Inputs=|+-
  Sum3 : Sum  Inputs=-+|
  Sum4 : Sum  Inputs=|+-
  Sum5 : Sum  Inputs=-+|
  Sum6 : Sum  Inputs=+-|
  Sum7 : Sum  Inputs=|-+
  To Workspace : ToWorkspace  VariableName=dp1  SampleTime=tsample
      settings: MaxDataPoints=Nsample
  To Workspace1 : ToWorkspace  VariableName=dp1m  SampleTime=tsample
      settings: MaxDataPoints=Nsample
  To Workspace10 : ToWorkspace  VariableName=v_track1_sim  SampleTime=tsample
      settings: MaxDataPoints=Nsample
  To Workspace11 : ToWorkspace  VariableName=v_track2_sim  SampleTime=tsample
      settings: MaxDataPoints=Nsample
  To Workspace12 : ToWorkspace  VariableName=v_track1_ref_sim  SampleTime=tsample
      settings: MaxDataPoints=Nsample
  To Workspace13 : ToWorkspace  VariableName=v_track2_ref_sim  SampleTime=tsample
      settings: MaxDataPoints=Nsample
  To Workspace2 : ToWorkspace  VariableName=ff_d1  SampleTime=tsample
      settings: MaxDataPoints=Nsample
  To Workspace3 : ToWorkspace  VariableName=dm1  SampleTime=tsample
      settings: MaxDataPoints=Nsample
  To Workspace4 : ToWorkspace  VariableName=ff_d2  SampleTime=tsample
      settings: MaxDataPoints=Nsample
  To Workspace5 : ToWorkspace  VariableName=dm1m  SampleTime=tsample
      settings: MaxDataPoints=Nsample
  To Workspace6 : ToWorkspace  VariableName=dp2  SampleTime=tsample
      settings: MaxDataPoints=Nsample
  To Workspace7 : ToWorkspace  VariableName=dp2m  SampleTime=tsample
      settings: MaxDataPoints=Nsample
  To Workspace8 : ToWorkspace  VariableName=dm2  SampleTime=tsample
      settings: MaxDataPoints=Nsample
  To Workspace9 : ToWorkspace  VariableName=dm2m  SampleTime=tsample
      settings: MaxDataPoints=Nsample
  Transfer Fcn : TransferFcn  Denominator=[1e-4 1]
  Transfer Fcn1 : TransferFcn  Denominator=[1e-4 1]
  Transfer Fcn2 : TransferFcn  Denominator=[2.5e-1 1]
  Transfer Fcn3 : TransferFcn  Denominator=[2.5e-1 1]
  direction : Subsystem
  direction_lineA : Subsystem
  direction_lineB : Subsystem
  direction_max_speed : Subsystem
  displacemets : Scope  NumInputPorts=4
  engine_load_compensation : Subsystem
  lineA_compensations : Subsystem
  "lineB_compensations " : Subsystem
  max_speed_limiter : Scope
  maximum_speed : Constant  Value=2
  omega_driver_gears : Scope
  pi_diff : Subsystem  mask{kp=kp_ctrl_diff_speed, ki=ki_ctrl_diff_speed, ts=tsample, sat_pos=(2-0.36)*2, sat_neg=-(2-0.36)*2}
  pi_sum : Subsystem  mask{kp=kp_ctrl_sum_speed, ki=ki_ctrl_sum_speed, ts=tsample, sat_pos=0 %(2-0.36)*2, sat_neg=-(2-0.36)*2}
  pressure_compensation : Subsystem
  tracking_diff : Scope
  tracking_speedA : Scope
  tracking_speed_B : Scope
  tracking_sum : Scope
  omegaA : PMIOPort  Side=Left
  omegaB : PMIOPort  Port=2  Side=Left
  tag scope: DmA=global, DmB=global, DpA=global, DpB=global, direction=global, omega_pu_m_A=global, omega_pu_m_B=global, pump_displacement_A=global, pump_displacement_B=global, steering_reference=global
  wires:
  Mux/1 -> tracking_diff/1
  [DpA] -> Mux1/1, To Workspace/1  "DpA"
  [DpAm] -> Mux1/2, To Workspace1/1  "DpAm"
  Mux2/1 -> displacemets/2
  [DmA] -> Mux2/1, To Workspace3/1  "DmA"
  [DmAm] -> Mux2/2, To Workspace5/1  "DmAm"
  Mux3/1 -> displacemets/3
  [DpB] -> Mux3/1, To Workspace6/1  "DpB"
  [DpBm] -> Mux3/2, To Workspace7/1  "DpBm"
  Mux4/1 -> displacemets/4
  [DmBm] -> Mux4/2, To Workspace9/1  "DmBm"
  [DmB] -> Mux4/1, To Workspace8/1  "DmB"
  [steering_reference] -> Mux/2, pi_diff/2(xref)  "w_diff_ref"
  Sum2/1 -> Gain1/1
  Gain3/1 -> Sum/1, Sum1/1, [omega_pu_m_A]
  Gain2/1 -> [omega_pu_m_B], Sum1/2, Sum/2  "omega_l_B"
  Sum3/1 -> Gain4/1
  Ap/1 -> [DpA], Abs1/1
  Bp/1 -> [DpB], Abs3/1
  Sum4/1 -> Sum6/2
  DmA_max/1 -> Sum6/1
  Sum6/1 -> Am/1
  Am/1 -> [DmA]
  DmB_max/1 -> Sum7/2
  Sum5/1 -> Sum7/1
  Sum7/1 -> Bm/1
  Bm/1 -> [DmB]
  Transfer Fcn1/1 -> Mux5/2, Gain8/1, Gain2/1  "omega_dgf_A"
  Transfer Fcn/1 -> Mux5/1, Gain3/1, Gain7/1  "omega_dgf_B"
  Mux5/1 -> omega_driver_gears/1
  Sum1/1 -> Mux/1, pi_diff/1(x)  "w_diff"
  Transfer Fcn2/1 -> Gain6/1
  Gain1/1 -> Sum8/1
  Gain4/1 -> Sum9/1
  Gain5/1 -> Sum8/2
  pi_sum/1(u) -> max_speed_limiter/1, Sum2/2, Sum3/2
  Sum/1 -> Abs4/1  "w_sum"
  Mux7/1 -> tracking_sum/1
  Transfer Fcn3/1 -> Gain5/1
  Constant/1 -> Manual Switch/1
  Constant1/1 -> Manual Switch/2
  Manual Switch/1 -> [direction]
  Abs/1 -> Sum4/1
  Abs1/1 -> Sum4/2
  Abs2/1 -> Sum5/2
  Abs3/1 -> Sum5/1
  Sum8/1 -> Sum10/2
  Sum9/1 -> Sum11/1
  maximum_speed/1 -> pi_sum/2(xref), Mux7/2  "w_sum_ref"
  [pump_displacement_A] -> direction_lineA/1(In1)
  [pump_displacement_B] -> direction_lineB/1(In1)
  Sum10/1 -> Abs/1, Ap/1
  Sum11/1 -> Abs2/1, Bp/1
  pi_diff/1(u) -> Sum3/1, Sum2/1
  Gain6/1 -> Sum9/2
  Subsystem1/1(Out1) -> To Workspace4/1, [pump_displacement_B]
  direction_lineA/1(Out1) -> Transfer Fcn3/1
  direction_lineB/1(Out1) -> Transfer Fcn2/1
  lineA_compensations/1(displacement_compensation) -> Sum10/1
  "lineB_compensations "/1(displacement_compensation) -> Sum11/2
  direction/1(Out1) -> [steering_reference]
  Mux1/1 -> displacemets/1
  Constant2/1 -> Sum13/1
  Constant3/1 -> Sum13/2
  Sum13/1 -> Gain11/1
  Mux6/1 -> tracking_speedA/1
  Gain7/1 -> To Workspace10/1, Mux6/1  "v_track1_sim"
  Constant4/1 -> Mux6/2, To Workspace12/1  "v_track1_ref_sim"
  Constant5/1 -> Mux8/2, To Workspace13/1  "v_track2_ref_sim"
  Gain8/1 -> To Workspace11/1, Mux8/1  "v_track2_sim"
  Mux8/1 -> tracking_speed_B/1
  PS-Simulink Converter5/1 -> Gain9/1
  Gain9/1 -> Transfer Fcn/1
  PS-Simulink Converter8/1 -> Gain10/1
  Gain10/1 -> Transfer Fcn1/1
  Gain11/1 -> direction/1(In1)
  Subsystem/1(Out1) -> To Workspace2/1, [pump_displacement_A]
  Abs4/1 -> Mux7/1, pi_sum/1(x)
  connections:
  PS-Simulink Converter5/LConn1 -- omegaA/RConn1
  omegaB/RConn1 -- PS-Simulink Converter8/LConn1

== system hdv_ctrl_2021_08_12/external_load/loadA ==
  Rate Limiter : RateLimiter  RisingSlewLimit=tau_load_max/2  FallingSlewLimit=-tau_load_max/2  SampleTimeMode=inherited
  Saturation : Saturate  UpperLimit=abs(tau_load)  LowerLimit=-abs(tau_load)
  Step : Step  Time=5  After=tau_load  SampleTime=0
  Out1 : Outport
  wires:
  Saturation/1 -> Out1/1
  Rate Limiter/1 -> Saturation/1
  Step/1 -> Rate Limiter/1

== system hdv_ctrl_2021_08_12/external_load/loadB ==
  Rate Limiter : RateLimiter  RisingSlewLimit=tau_load_max/2  FallingSlewLimit=-tau_load_max/2  SampleTimeMode=inherited
  Saturation : Saturate  UpperLimit=abs(tau_load)  LowerLimit=-abs(tau_load)
  Step : Step  Time=5  After=tau_load  SampleTime=0
  Out1 : Outport
  wires:
  Step/1 -> Rate Limiter/1
  Rate Limiter/1 -> Saturation/1
  Saturation/1 -> Out1/1

== system hdv_ctrl_2021_08_12/vehicle_speed_control/Subsystem ==
  Sum12 : Sum  Inputs=++-
  Transfer Fcn : TransferFcn  Denominator=[1 1]
  feed_forward_A : Step  Time=5  After=d1_ff  SampleTime=0
  feed_forward_A1 : Step  Time=simulation_length/3  After=d1_ff  SampleTime=0
  feed_forward_A2 : Step  Time=simulation_length/3*2  After=d1_ff  SampleTime=0
  Out1 : Outport
  wires:
  Sum12/1 -> Transfer Fcn/1
  feed_forward_A/1 -> Sum12/2
  Transfer Fcn/1 -> Out1/1
  feed_forward_A2/1 -> Sum12/1
  feed_forward_A1/1 -> Sum12/3

== system hdv_ctrl_2021_08_12/vehicle_speed_control/Subsystem1 ==
  Sum12 : Sum  Inputs=++-
  Transfer Fcn : TransferFcn  Denominator=[1 1]
  feed_forward_B : Step  Time=5  After=d2_ff  SampleTime=0
  feed_forward_B1 : Step  Time=simulation_length/3  After=d2_ff  SampleTime=0
  feed_forward_B2 : Step  Time=simulation_length/3*2  After=d2_ff  SampleTime=0
  Out1 : Outport
  wires:
  feed_forward_B/1 -> Sum12/2
  Sum12/1 -> Transfer Fcn/1
  Transfer Fcn/1 -> Out1/1
  feed_forward_B2/1 -> Sum12/1
  feed_forward_B1/1 -> Sum12/3

== system hdv_ctrl_2021_08_12/vehicle_speed_control/direction ==
  In1 : Inport
  Product : Product
  Out1 : Outport
  wires:
  [direction] -> Product/2
  In1/1 -> Product/1
  Product/1 -> Out1/1

== system hdv_ctrl_2021_08_12/vehicle_speed_control/direction_lineA ==
  In1 : Inport
  Product : Product
  Out1 : Outport
  wires:
  Product/1 -> Out1/1
  In1/1 -> Product/1
  [direction] -> Product/2

== system hdv_ctrl_2021_08_12/vehicle_speed_control/direction_lineB ==
  In1 : Inport
  Product : Product
  Out1 : Outport
  wires:
  [direction] -> Product/2
  In1/1 -> Product/1
  Product/1 -> Out1/1

== system hdv_ctrl_2021_08_12/vehicle_speed_control/direction_max_speed ==
  In1 : Inport
  Product : Product
  Out1 : Outport
  wires:
  Product/1 -> Out1/1
  In1/1 -> Product/1
  [direction] -> Product/2

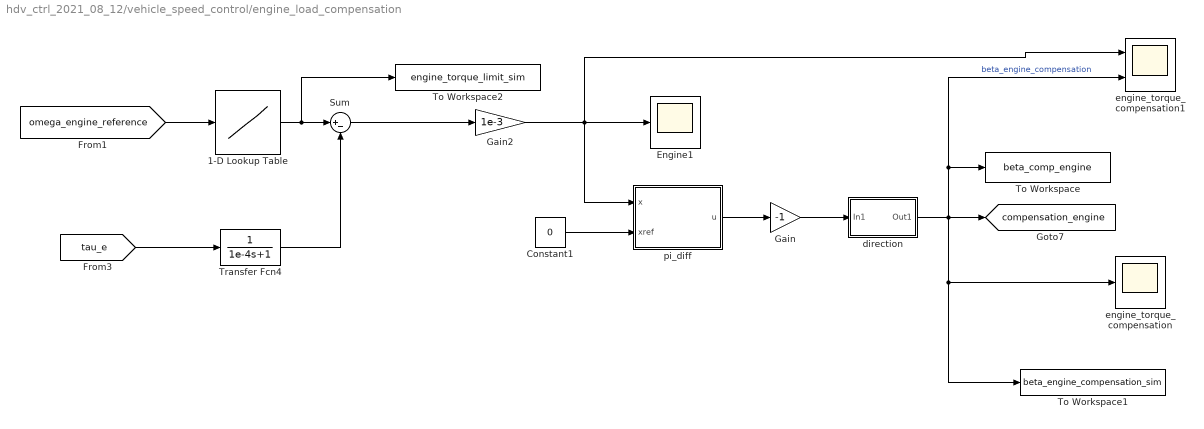
== system hdv_ctrl_2021_08_12/vehicle_speed_control/engine_load_compensation ==
  1-D Lookup Table : Lookup_n-D  NumberOfTableDimensions=1  BreakpointsForDimension1=rpm  Table=available_torque  InternalRulePriority=Speed  RndMeth=Simplest  InputSameDT=on
  Constant1 : Constant  Value=0
  Engine1 : Scope
  Gain : Gain  Gain=-1
  Gain2 : Gain  Gain=1e-3
  Sum : Sum  Inputs=|+-
  To Workspace : ToWorkspace  VariableName=beta_comp_engine  SampleTime=tsample
      settings: MaxDataPoints=Nsample
  To Workspace1 : ToWorkspace  VariableName=beta_engine_compensation_sim  SampleTime=tsample
      settings: MaxDataPoints=Nsample
  To Workspace2 : ToWorkspace  VariableName=engine_torque_limit_sim  SampleTime=tsample
      settings: MaxDataPoints=Nsample
  Transfer Fcn4 : TransferFcn  Denominator=[1e-4 1]
  direction : Subsystem
  engine_torque_compensation : Scope
  engine_torque_compensation1 : Scope  NumInputPorts=2
  pi_diff : Subsystem  mask{kp=1.25, ki=2.5, ts=tsample, sat_pos=(2-0.36), sat_neg=0}
  tag scope: compensation_engine=global
  wires:
  Transfer Fcn4/1 -> Sum/2
  1-D Lookup Table/1 -> To Workspace2/1, Sum/1
  pi_diff/1(u) -> Gain/1
  [omega_engine_reference] -> 1-D Lookup Table/1
  [tau_e] -> Transfer Fcn4/1
  Constant1/1 -> pi_diff/2(xref)
  Gain/1 -> direction/1(In1)
  direction/1(Out1) -> engine_torque_compensation1/2, To Workspace/1, To Workspace1/1, engine_torque_compensation/1, [compensation_engine]  "beta_engine_compensation"
  Sum/1 -> Gain2/1
  Gain2/1 -> engine_torque_compensation1/1, pi_diff/1(x), Engine1/1

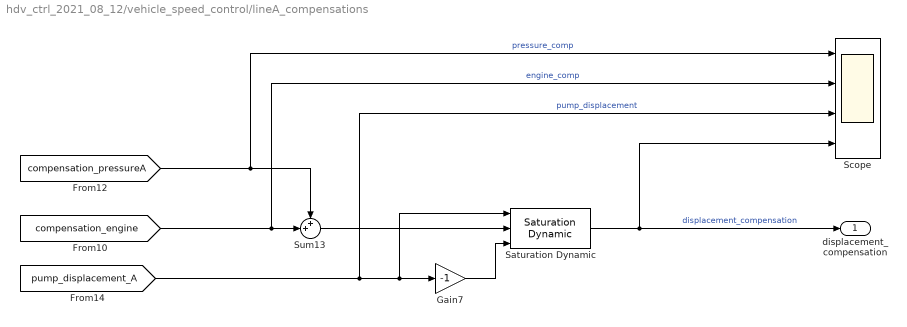
== system hdv_ctrl_2021_08_12/vehicle_speed_control/lineA_compensations ==
  Gain7 : Gain  Gain=-1
  Saturation Dynamic : simulink/Discontinuities/Saturation Dynamic  OutMin=[]  OutMax=[]  OutDataTypeStr=Inherit: Same as second input  OutDataType=fixdt(1, 16)  OutScaling=2^-10  DoSatur=off
  Scope : Scope  NumInputPorts=4
  Sum13 : Sum  Inputs=++|
  displacement_compensation : Outport
  wires:
  [pump_displacement_A] -> Scope/3, Saturation Dynamic/1, Gain7/1  "pump_displacement"
  Saturation Dynamic/1 -> Scope/4, displacement_compensation/1  "displacement_compensation"
  Sum13/1 -> Saturation Dynamic/2
  [compensation_engine] -> Scope/2, Sum13/2  "engine_comp"
  Gain7/1 -> Saturation Dynamic/3
  [compensation_pressureA] -> Scope/1, Sum13/1  "pressure_comp"

== system hdv_ctrl_2021_08_12/vehicle_speed_control/lineB_compensations  ==
  Gain7 : Gain  Gain=-1
  Saturation Dynamic : simulink/Discontinuities/Saturation Dynamic  OutMin=[]  OutMax=[]  OutDataTypeStr=Inherit: Same as second input  OutDataType=fixdt(1, 16)  OutScaling=2^-10  DoSatur=off
  Sum12 : Sum  Inputs=|++
  displacement_compensation : Outport
  wires:
  [compensation_engine] -> Sum12/1
  [compensation_pressureB] -> Sum12/2
  Gain7/1 -> Saturation Dynamic/3
  Sum12/1 -> Saturation Dynamic/2
  [pump_displacement_B] -> Saturation Dynamic/1, Gain7/1
  Saturation Dynamic/1 -> displacement_compensation/1

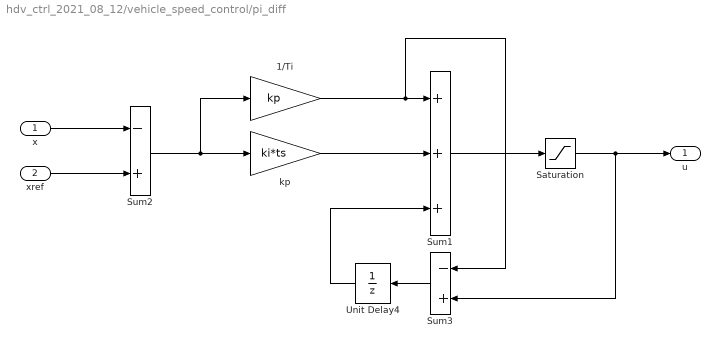
== system hdv_ctrl_2021_08_12/vehicle_speed_control/pi_diff ==
  x : Inport
  xref : Inport  Port=2
  1/Ti : Gain  Gain=kp  SaturateOnIntegerOverflow=on  OutDataTypeStr=Inherit: Same as input  ParamDataTypeStr=Inherit: Same as input
  Saturation : Saturate  UpperLimit=sat_pos  LowerLimit=sat_neg
  Sum1 : Sum  Inputs=+++  SaturateOnIntegerOverflow=on
  Sum2 : Sum  Inputs=-+  SaturateOnIntegerOverflow=on
  Sum3 : Sum  Inputs=-+  SaturateOnIntegerOverflow=on
  Unit Delay4 : UnitDelay  SampleTime=ts  HasFrameUpgradeWarning=on
  kp : Gain  Gain=ki*ts  SaturateOnIntegerOverflow=on  OutDataTypeStr=Inherit: Same as input  ParamDataTypeStr=Inherit: Same as input
  u : Outport
  wires:
  Saturation/1 -> Sum3/2, u/1
  Unit Delay4/1 -> Sum1/3
  Sum1/1 -> Saturation/1
  x/1 -> Sum2/1
  Sum3/1 -> Unit Delay4/1
  1/Ti/1 -> Sum3/1, Sum1/1
  Sum2/1 -> 1/Ti/1, kp/1
  kp/1 -> Sum1/2
  xref/1 -> Sum2/2

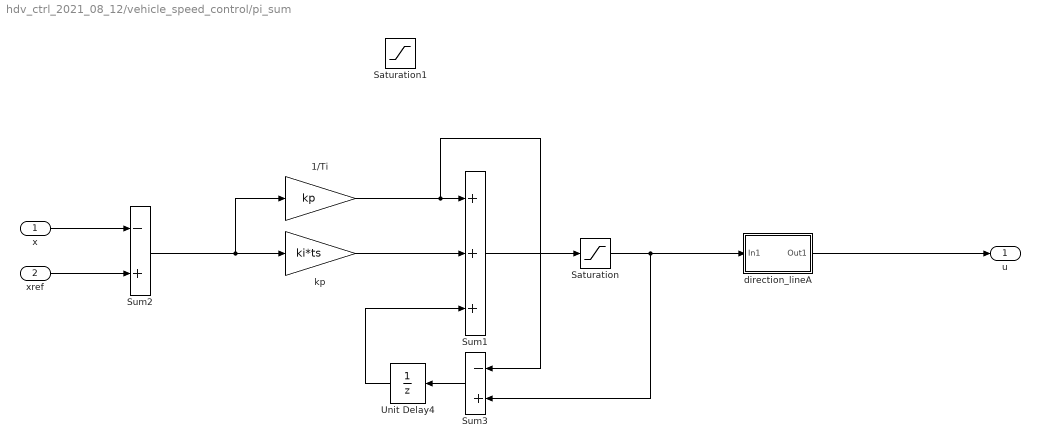
== system hdv_ctrl_2021_08_12/vehicle_speed_control/pi_sum ==
  x : Inport
  xref : Inport  Port=2
  1/Ti : Gain  Gain=kp  SaturateOnIntegerOverflow=on  OutDataTypeStr=Inherit: Same as input  ParamDataTypeStr=Inherit: Same as input
  Saturation : Saturate  UpperLimit=sat_pos  LowerLimit=sat_neg
  Saturation1 : Saturate  UpperLimit=0  LowerLimit=-inf
  Sum1 : Sum  Inputs=+++  SaturateOnIntegerOverflow=on
  Sum2 : Sum  Inputs=-+  SaturateOnIntegerOverflow=on
  Sum3 : Sum  Inputs=-+  SaturateOnIntegerOverflow=on
  Unit Delay4 : UnitDelay  SampleTime=ts  HasFrameUpgradeWarning=on
  direction_lineA : Subsystem
  kp : Gain  Gain=ki*ts  SaturateOnIntegerOverflow=on  OutDataTypeStr=Inherit: Same as input  ParamDataTypeStr=Inherit: Same as input
  u : Outport
  wires:
  xref/1 -> Sum2/2
  kp/1 -> Sum1/2
  1/Ti/1 -> Sum1/1, Sum3/1
  Sum3/1 -> Unit Delay4/1
  x/1 -> Sum2/1
  Sum1/1 -> Saturation/1
  Unit Delay4/1 -> Sum1/3
  Saturation/1 -> direction_lineA/1(In1), Sum3/2
  Sum2/1 -> kp/1, 1/Ti/1
  direction_lineA/1(Out1) -> u/1

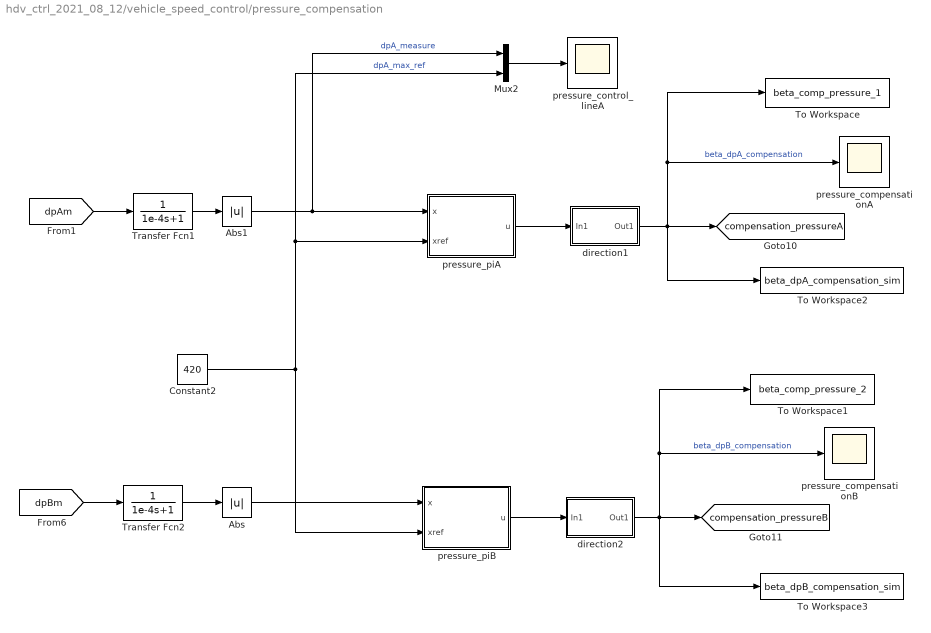
== system hdv_ctrl_2021_08_12/vehicle_speed_control/pressure_compensation ==
  Abs : Abs
  Abs1 : Abs
  Constant2 : Constant  Value=420
  Mux2 : Mux  Inputs=2
  To Workspace : ToWorkspace  VariableName=beta_comp_pressure_1  SampleTime=tsample
      settings: MaxDataPoints=Nsample
  To Workspace1 : ToWorkspace  VariableName=beta_comp_pressure_2  SampleTime=tsample
      settings: MaxDataPoints=Nsample
  To Workspace2 : ToWorkspace  VariableName=beta_dpA_compensation_sim  SampleTime=tsample
      settings: MaxDataPoints=Nsample
  To Workspace3 : ToWorkspace  VariableName=beta_dpB_compensation_sim  SampleTime=tsample
      settings: MaxDataPoints=Nsample
  Transfer Fcn1 : TransferFcn  Denominator=[1e-4 1]
  Transfer Fcn2 : TransferFcn  Denominator=[1e-4 1]
  direction1 : Subsystem
  direction2 : Subsystem
  pressure_compensationA : Scope
  pressure_compensationB : Scope
  pressure_control_lineA : Scope
  pressure_piA : Subsystem  mask{kp=0.0025, ki=0.02, ts=tsample, sat_pos=0, sat_neg=-(2-0.36)}
  pressure_piB : Subsystem  mask{kp=0.0025, ki=0.02, ts=tsample, sat_pos=0, sat_neg=-(2-0.36)}
  tag scope: compensation_pressureA=global, compensation_pressureB=global
  wires:
  Abs1/1 -> pressure_piA/1(x), Mux2/1  "dpA_measure"
  Transfer Fcn1/1 -> Abs1/1
  [dpBm] -> Transfer Fcn2/1
  Constant2/1 -> pressure_piB/2(xref), pressure_piA/2(xref), Mux2/2  "dpA_max_ref"
  Abs/1 -> pressure_piB/1(x)
  direction1/1(Out1) -> To Workspace2/1, To Workspace/1, pressure_compensationA/1, [compensation_pressureA]  "beta_dpA_compensation"
  Mux2/1 -> pressure_control_lineA/1
  [dpAm] -> Transfer Fcn1/1
  pressure_piB/1(u) -> direction2/1(In1)
  direction2/1(Out1) -> To Workspace3/1, [compensation_pressureB], To Workspace1/1, pressure_compensationB/1  "beta_dpB_compensation"
  Transfer Fcn2/1 -> Abs/1
  pressure_piA/1(u) -> direction1/1(In1)

== system hdv_ctrl_2021_08_12/vehicle_speed_control/engine_load_compensation/direction ==
  In1 : Inport
  Product : Product
  Out1 : Outport
  wires:
  Product/1 -> Out1/1
  In1/1 -> Product/1
  [direction] -> Product/2

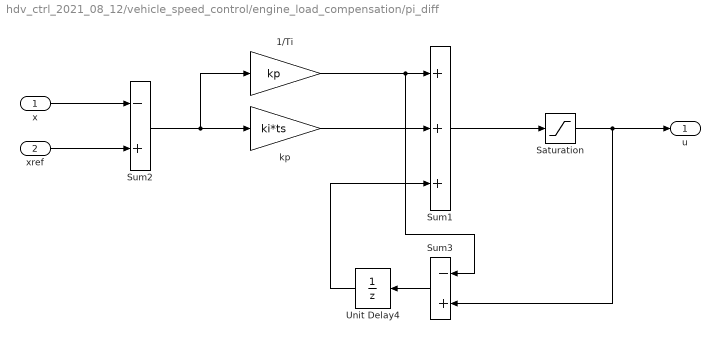
== system hdv_ctrl_2021_08_12/vehicle_speed_control/engine_load_compensation/pi_diff ==
  x : Inport
  xref : Inport  Port=2
  1/Ti : Gain  Gain=kp  SaturateOnIntegerOverflow=on  OutDataTypeStr=Inherit: Same as input  ParamDataTypeStr=Inherit: Same as input
  Saturation : Saturate  UpperLimit=sat_pos  LowerLimit=sat_neg
  Sum1 : Sum  Inputs=+++  SaturateOnIntegerOverflow=on
  Sum2 : Sum  Inputs=-+  SaturateOnIntegerOverflow=on
  Sum3 : Sum  Inputs=-+  SaturateOnIntegerOverflow=on
  Unit Delay4 : UnitDelay  SampleTime=ts  HasFrameUpgradeWarning=on
  kp : Gain  Gain=ki*ts  SaturateOnIntegerOverflow=on  OutDataTypeStr=Inherit: Same as input  ParamDataTypeStr=Inherit: Same as input
  u : Outport
  wires:
  Saturation/1 -> u/1, Sum3/2
  Unit Delay4/1 -> Sum1/3
  Sum1/1 -> Saturation/1
  x/1 -> Sum2/1
  Sum3/1 -> Unit Delay4/1
  1/Ti/1 -> Sum3/1, Sum1/1
  Sum2/1 -> 1/Ti/1, kp/1
  kp/1 -> Sum1/2
  xref/1 -> Sum2/2

== system hdv_ctrl_2021_08_12/vehicle_speed_control/pi_sum/direction_lineA ==
  In1 : Inport
  Product : Product
  Out1 : Outport
  wires:
  Product/1 -> Out1/1
  In1/1 -> Product/1
  [direction] -> Product/2

== system hdv_ctrl_2021_08_12/vehicle_speed_control/pressure_compensation/direction1 ==
  In1 : Inport
  Product : Product
  Out1 : Outport
  wires:
  [direction] -> Product/2
  In1/1 -> Product/1
  Product/1 -> Out1/1

== system hdv_ctrl_2021_08_12/vehicle_speed_control/pressure_compensation/direction2 ==
  In1 : Inport
  Product : Product
  Out1 : Outport
  wires:
  Product/1 -> Out1/1
  In1/1 -> Product/1
  [direction] -> Product/2

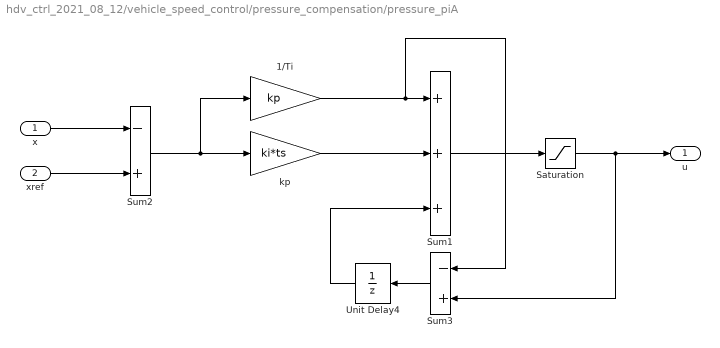
== system hdv_ctrl_2021_08_12/vehicle_speed_control/pressure_compensation/pressure_piA ==
  x : Inport
  xref : Inport  Port=2
  1/Ti : Gain  Gain=kp  SaturateOnIntegerOverflow=on  OutDataTypeStr=Inherit: Same as input  ParamDataTypeStr=Inherit: Same as input
  Saturation : Saturate  UpperLimit=sat_pos  LowerLimit=sat_neg
  Sum1 : Sum  Inputs=+++  SaturateOnIntegerOverflow=on
  Sum2 : Sum  Inputs=-+  SaturateOnIntegerOverflow=on
  Sum3 : Sum  Inputs=-+  SaturateOnIntegerOverflow=on
  Unit Delay4 : UnitDelay  SampleTime=ts  HasFrameUpgradeWarning=on
  kp : Gain  Gain=ki*ts  SaturateOnIntegerOverflow=on  OutDataTypeStr=Inherit: Same as input  ParamDataTypeStr=Inherit: Same as input
  u : Outport
  wires:
  xref/1 -> Sum2/2
  kp/1 -> Sum1/2
  Sum2/1 -> kp/1, 1/Ti/1
  1/Ti/1 -> Sum1/1, Sum3/1
  Sum3/1 -> Unit Delay4/1
  x/1 -> Sum2/1
  Sum1/1 -> Saturation/1
  Unit Delay4/1 -> Sum1/3
  Saturation/1 -> u/1, Sum3/2

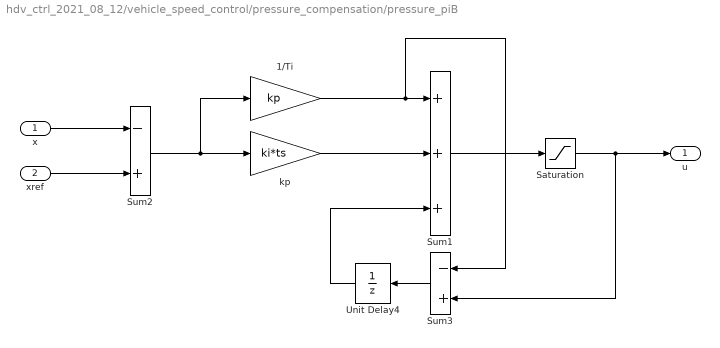
== system hdv_ctrl_2021_08_12/vehicle_speed_control/pressure_compensation/pressure_piB ==
  x : Inport
  xref : Inport  Port=2
  1/Ti : Gain  Gain=kp  SaturateOnIntegerOverflow=on  OutDataTypeStr=Inherit: Same as input  ParamDataTypeStr=Inherit: Same as input
  Saturation : Saturate  UpperLimit=sat_pos  LowerLimit=sat_neg
  Sum1 : Sum  Inputs=+++  SaturateOnIntegerOverflow=on
  Sum2 : Sum  Inputs=-+  SaturateOnIntegerOverflow=on
  Sum3 : Sum  Inputs=-+  SaturateOnIntegerOverflow=on
  Unit Delay4 : UnitDelay  SampleTime=ts  HasFrameUpgradeWarning=on
  kp : Gain  Gain=ki*ts  SaturateOnIntegerOverflow=on  OutDataTypeStr=Inherit: Same as input  ParamDataTypeStr=Inherit: Same as input
  u : Outport
  wires:
  Saturation/1 -> Sum3/2, u/1
  Unit Delay4/1 -> Sum1/3
  Sum1/1 -> Saturation/1
  x/1 -> Sum2/1
  Sum3/1 -> Unit Delay4/1
  1/Ti/1 -> Sum3/1, Sum1/1
  Sum2/1 -> 1/Ti/1, kp/1
  kp/1 -> Sum1/2
  xref/1 -> Sum2/2
